simulink model "PIDctrl"  (R2020b)
settings: Solver=VariableStepAuto  StartTime=0.0  StopTime=0.2  RelTol=1e-3
values from neighbouring files (symbols this model uses):
  Ki = 500.0    [Problem4_data.sldd]
  Kp = 50.0    [Problem4_data.sldd]
  Ts = 0.0001    [Problem4_data.sldd]
settings Model: DataDictionary=Problem4_data.sldd  Creator=ASUS  LastModifiedBy=ASUS
settings SolverCC: AlgebraicLoopSolver=LineSearch
settings DataIOCC: SaveOutput=off  SaveTime=off

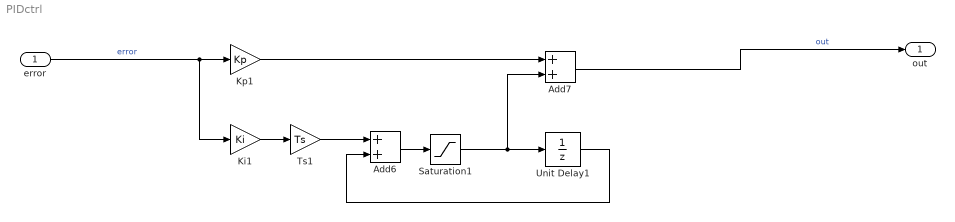
== system PIDctrl ==
  error : Inport  OutDataTypeStr=double  PortDimensions=1  SampleTime=0
  Add6 : Sum
  Add7 : Sum
  Ki1 : Gain  Gain=Ki
  Kp1 : Gain  Gain=Kp
  Saturation1 : Saturate  UpperLimit=1  LowerLimit=-1
  Ts1 : Gain  Gain=Ts
  Unit Delay1 : UnitDelay  SampleTime=-1  HasFrameUpgradeWarning=on
  out : Outport  OutDataTypeStr=double  PortDimensions=1  SampleTime=0
  wires:
  Saturation1/1 -> Add7/2, Unit Delay1/1
  Kp1/1 -> Add7/1
  error/1 -> Kp1/1, Ki1/1  "error"
  Ki1/1 -> Ts1/1
  Add6/1 -> Saturation1/1
  Ts1/1 -> Add6/1
  Unit Delay1/1 -> Add6/2
  Add7/1 -> out/1  "out"
